simulink model "untitled"  (R2025b)
settings: Solver=FixedStepDiscrete  StartTime=0.0  StopTime=inf  FixedStep=0.01  RelTol=1e-3
libraries: instrumentseriallib x2
settings Model: Creator=chromatedkid  LastModifiedBy=chromatedkid
settings OptimizationCC: DefaultParameterBehavior=Inlined  EnhancedBackFolding=on  PassReuseOutputArgsAs=Individual arguments  ZeroExternalMemoryAtStartup=off  ZeroInternalMemoryAtStartup=off  OptimizeBlockOrder=speed  DifferentSizesBufferReuse=on  OptimizationCustomize=off  EfficientTunableParamExpr=on
settings DebuggingCC: ParameterTunabilityLossMsg=error
settings HardwareCC: ProdBitPerPointer=32.0  ProdBitPerSizeT=32.0  ProdBitPerPtrDiffT=32.0  ProdWordSize=32.0  ProdLongLongMode=on  ProdHWDeviceType=RISC-V->RV32I
settings SFSimCC: MATLABDynamicMemAlloc=off  SimTargetLang=C++  SimDLTargetLibrary=mkl-dnn
settings RTWCC: SystemTargetFile=ert.tlc  GenCodeOnly=on  TemplateMakefile=ert_default_tmf  TargetLang=C++  Description=Embedded Coder
settings CodeAppCC: ForceParamTrailComments=on  IgnoreCustomStorageClasses=off  OperatorAnnotations=on  SimulinkDataObjDesc=on  SFDataObjDesc=on  InsertBlockDesc=on
settings ERTTargetCC: RootIOFormat=Structure reference  ERTCustomFileTemplate=example_file_process.tlc  ERTFilePackagingFormat=Compact  TargetLangStandard=C++20 (ISO)  GenerateSampleERTMain=on  CodeInterfacePackaging=C++ class  SubcomponentCodeInterfacePackaging=C++ class

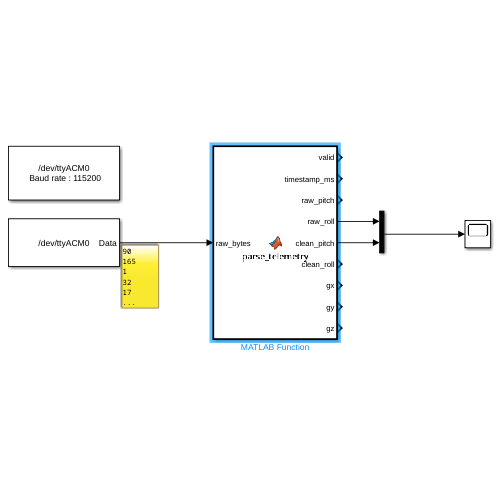
[thumbnail: Simulink's stored preview of the top-level diagram]
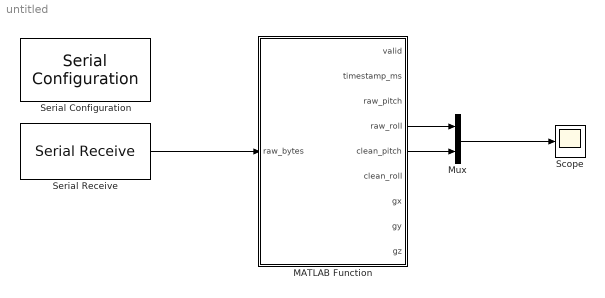
== system untitled ==
  MATLAB Function : MATLAB Function  TreatAsAtomicUnit=on
  Mux : Mux  Inputs=2
  Scope : Scope
      settings: ActiveDisplayYMinimum=-105.51357380726434  ActiveDisplayYMaximum=173.26034840938144
  Serial Configuration : instrumentseriallib/Serial Configuration  Priority=-200000  PortSel=/dev/ttyACM0  Port=/dev/ttyACM0  ComPort=/dev/ttyACM0  BaudRate=115200  DataBits=8  Parity=none  StopBits=1  ByteOrder=little-endian  FlowControl=none  Timeout=10  SimulateUsing=Interpreted execution  BlockInModel=on  aMode=1
      settings: LibrarySourceBlock=embeddedtargetslib/Host Communication/Serial Configuration
  Serial Receive : instrumentseriallib/Serial Receive  Priority=1  PortSel=/dev/ttyACM0  Port=/dev/ttyACM0  ComPort=/dev/ttyACM0  DataType=uint8  SaveDataType=uint8  ToggleHeader=off  Header=[170 85]  ToggleDataSize=on  DataSize=[38 1]  ToggleTerminator=off  Terminator=Custom terminator  CustomTerminator=[10]  InputFormat=Column major  EnableBlockingMode=on  ActionDataUnavailable=Output last received value  ActionWhenDataUnavailable=Output last received value  CustomValue=0  SampleTime=0.01  SimulateUsing=Interpreted execution  BlockInModel=on  aMode=1  LibraryInUse=instrumentlib
  wires:
  Serial Receive/1 -> MATLAB Function/1(raw_bytes)
  MATLAB Function/4(raw_roll) -> Mux/1
  MATLAB Function/5(clean_pitch) -> Mux/2
  Mux/1 -> Scope/1

== matlab function untitled/MATLAB Function ==
  data: raw_bytes input; valid output; timestamp_ms output; raw_pitch output; raw_roll output; clean_pitch output; clean_roll output; gx output; gy output; gz output
function [valid, timestamp_ms, raw_pitch, raw_roll, clean_pitch, clean_roll, gx, gy, gz] = parse_telemetry(raw_bytes)

persistent state rx_buf rx_idx expected_len msg_id crc_low
if isempty(state)
    state        = uint8(0);
    rx_buf       = uint8(zeros(1, 64));
    rx_idx       = uint32(1);
    expected_len = uint8(0);
    msg_id       = uint8(0);
    crc_low      = uint8(0);
end

valid        = false;
timestamp_ms = uint32(0);
raw_pitch    = single(0);
raw_roll     = single(0);
clean_pitch  = single(0);
clean_roll   = single(0);
gx           = single(0);
gy           = single(0);
gz           = single(0);

for i = 1:length(raw_bytes)
    % Принудительное приведение каждого байта к uint8
    b = uint8(raw_bytes(i));

    switch state
        case 0 % SYNC_LOW (0x5A)
            if b == uint8(90) % 0x5A
                state = uint8(1);
            end

        case 1 % SYNC_HIGH (0xA5)
            if b == uint8(165) % 0xA5
                state = uint8(2);
            else
                state = uint8(0);
            end

        case 2 % MSG_ID
            msg_id = b;
            state  = uint8(3);

        case 3 % LENGTH
            if b <= uint8(64)
                expected_len = b;
                rx_idx       = uint32(1);
                if expected_len > uint8(0)
                    state = uint8(4);
                else
                    state = uint8(5);
                end
            else
                state = uint8(0);
            end

        case 4 % PAYLOAD
            rx_buf(rx_idx) = b;
            rx_idx = rx_idx + uint32(1);
            if rx_idx > uint32(expected_len)
                state = uint8(5);
            end

        case 5 % CRC16 LOW
            crc_low = b;
            state   = uint8(6);

        case 6 % CRC16 HIGH & Проверка
            crc_high = b;
            crc_received = bitor(uint16(crc_low), bitshift(uint16(crc_high), 8));
            state = uint8(0);

            % Расчет контрольной суммы от ID, LEN и полезной нагрузки
            len_double = double(expected_len);
            calc_data = [msg_id, expected_len, rx_buf(1:len_double)];
            crc_calc = uint16(65535);

            for k = 1:length(calc_data)
                crc_calc = bitxor(crc_calc, bitshift(uint16(calc_data(k)), 8));
                for bit = 1:8
                    if bitand(crc_calc, uint16(32768)) ~= 0
                        crc_calc = bitxor(bitshift(crc_calc, 1), uint16(4129));
                    else
                        crc_calc = bitshift(crc_calc, 1);
                    end
                end
            end

            if (crc_calc == crc_received) && (msg_id == uint8(1)) && (expected_len == uint8(32))
                timestamp_ms = typecast(rx_buf(1:4),   'uint32');
                raw_pitch    = typecast(rx_buf(5:8),   'single');
                raw_roll     = typecast(rx_buf(9:12),  'single');
                clean_pitch  = typecast(rx_buf(13:16), 'single');
                clean_roll   = typecast(rx_buf(17:20), 'single');
                gx           = typecast(rx_buf(21:24), 'single');
                gy           = typecast(rx_buf(25:28), 'single');
                gz           = typecast(rx_buf(29:32), 'single');
                valid        = true;
            end
    end
end
